simulink model "mod342_3"  (R2024b)
settings: Solver=ode45  StartTime=0.0  StopTime=9999  MaxStep=.01  RelTol=1e-3  AbsTol=1e-6
libraries: simulink x1
settings Model: Creator=vise  LastModifiedBy=Xist
settings DataIOCC: SaveFormat=Array  SignalLoggingSaveFormat=ModelDataLogs  ReturnWorkspaceOutputs=off
settings OptimizationCC: BooleanDataType=off
settings DebuggingCC: SaveWithParameterizedLinksMsg=none  UnderspecifiedInitializationDetection=Classic  MergeDetectMultiDrivingBlocksExec=none  SignalResolutionControl=TryResolveAllWithWarning  MultiTaskDSMMsg=warning  MultiTaskCondExecSysMsg=none  UnconnectedInputMsg=warning  UnconnectedOutputMsg=warning  UnconnectedLineMsg=warning
settings HardwareCC: TargetUnknown=on
settings ModelReferenceCC: PropagateSignalLabelsOutOfModel=off
settings RTWCC: TemplateMakefile=grt_unix.tmf
settings GRTTargetCC: CombineOutputUpdateFcns=off  GRTInterface=on
settings ConfigComp: CovMetricSettings=dw

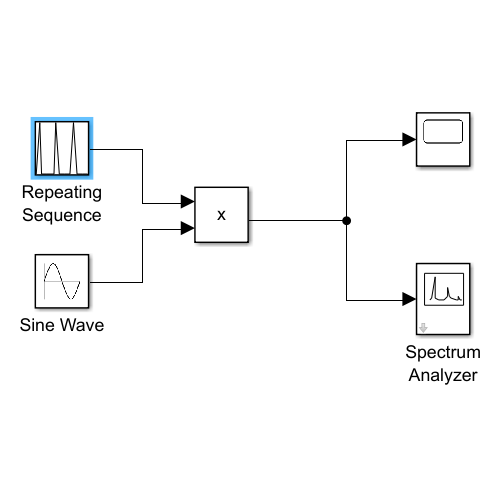
[thumbnail: Simulink's stored preview of the top-level diagram]
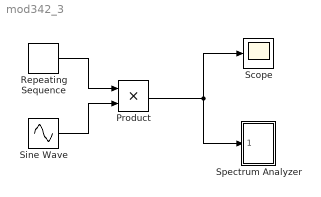
== system mod342_3 ==
  Product : Product  InputSameDT=on  RndMeth=Zero  SaturateOnIntegerOverflow=on  OutDataTypeStr=Inherit: Same as first input
  Repeating Sequence : simulink/Sources/Repeating Sequence  rep_seq_t=[0 0.5 1 2 3]  rep_seq_y=[0 1 0 0 0]
      settings: LibrarySourceBlock=|
      | simulink3/Sources/Repeating
      | Sequence
  Scope : Scope
  Sine Wave : Sin  Frequency=2*pi*10  SampleTime=0
  Spectrum Analyzer : Subsystem  mask(Spectrum analyzer.){N=2048, T_s=0.02, plot_period=10}
      mask prompts: N "Number of sample points:"; T_s "Sampling period (sec):"; plot_period "Plotting Period (sec):"
      mask Help: EE438 Lab utility; See Prof. Bouman.
      mask Display: plot(0,0,100,100,[14,91,91,14,14],[86,86,40,40,86],[85,82,80,79,75,67,63,60,57,53,41,36,33,27,24],[49,50,53,50,49,51,54,66,54,50,50,52,81,51,49])
  wires:
  Product/1 -> Spectrum Analyzer/1(input signal), Scope/1
  Repeating Sequence/1 -> Product/1
  Sine Wave/1 -> Product/2

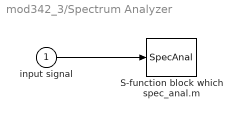
== system mod342_3/Spectrum Analyzer ==
  input signal : Inport
  S-function block which spec_anal.m : S-Function  FunctionName=SpecAnal  Parameters=N,T_s,plot_period  SFunctionDeploymentMode=off  EnableBusSupport=off
  wires:
  input signal/1 -> S-function block which spec_anal.m/1
